simulink subsystem "Pack_SOC_Estimation"  (R2021a)
settings: Solver=VariableStepAuto  StartTime=0.0  StopTime=10.0  RelTol=1e-3
(part 2 of 4)

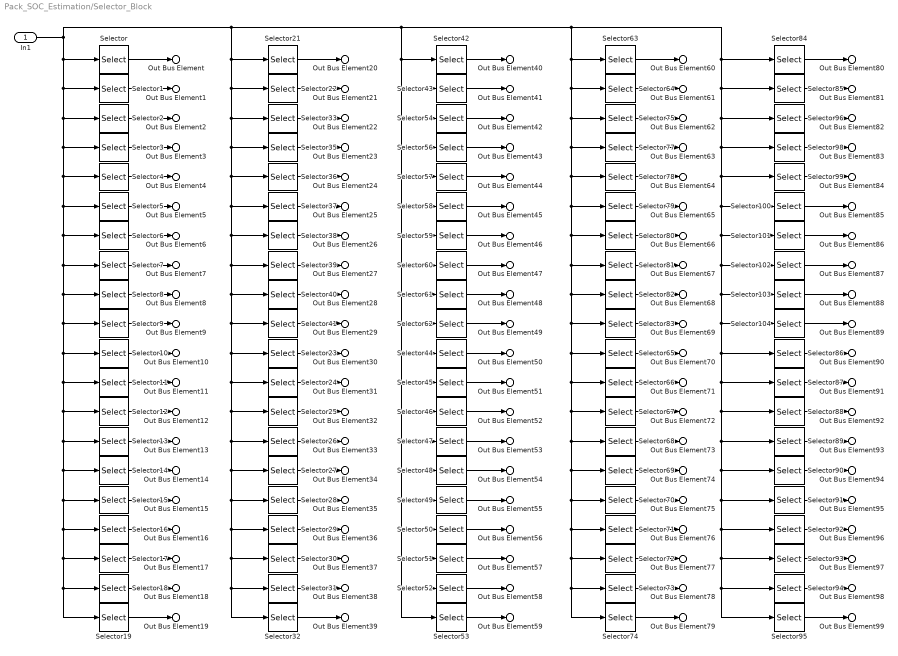
== system Pack_SOC_Estimation/Selector_Block ==
  In1 : Inport
  Selector : Selector  NumberOfDimensions=2  InputPortWidth=3  IndexOptions=Index vector (dialog),Index vector (dialog)  Indices=1,1  OutputSizes=1,1
  Selector1 : Selector  NumberOfDimensions=2  InputPortWidth=3  IndexOptions=Index vector (dialog),Index vector (dialog)  Indices=1,2  OutputSizes=1,1
  Selector10 : Selector  NumberOfDimensions=2  InputPortWidth=3  IndexOptions=Index vector (dialog),Index vector (dialog)  Indices=2,1  OutputSizes=1,1
  Selector100 : Selector  NumberOfDimensions=2  InputPortWidth=3  IndexOptions=Index vector (dialog),Index vector (dialog)  Indices=9,6  OutputSizes=1,1
  Selector101 : Selector  NumberOfDimensions=2  InputPortWidth=3  IndexOptions=Index vector (dialog),Index vector (dialog)  Indices=9,7  OutputSizes=1,1
  Selector102 : Selector  NumberOfDimensions=2  InputPortWidth=3  IndexOptions=Index vector (dialog),Index vector (dialog)  Indices=9,8  OutputSizes=1,1
  Selector103 : Selector  NumberOfDimensions=2  InputPortWidth=3  IndexOptions=Index vector (dialog),Index vector (dialog)  Indices=9,9  OutputSizes=1,1
  Selector104 : Selector  NumberOfDimensions=2  InputPortWidth=3  IndexOptions=Index vector (dialog),Index vector (dialog)  Indices=9,10  OutputSizes=1,1
  Selector11 : Selector  NumberOfDimensions=2  InputPortWidth=3  IndexOptions=Index vector (dialog),Index vector (dialog)  Indices=2,2  OutputSizes=1,1
  Selector12 : Selector  NumberOfDimensions=2  InputPortWidth=3  IndexOptions=Index vector (dialog),Index vector (dialog)  Indices=2,3  OutputSizes=1,1
  Selector13 : Selector  NumberOfDimensions=2  InputPortWidth=3  IndexOptions=Index vector (dialog),Index vector (dialog)  Indices=2,4  OutputSizes=1,1
  Selector14 : Selector  NumberOfDimensions=2  InputPortWidth=3  IndexOptions=Index vector (dialog),Index vector (dialog)  Indices=2,5  OutputSizes=1,1
  Selector15 : Selector  NumberOfDimensions=2  InputPortWidth=3  IndexOptions=Index vector (dialog),Index vector (dialog)  Indices=2,6  OutputSizes=1,1
  Selector16 : Selector  NumberOfDimensions=2  InputPortWidth=3  IndexOptions=Index vector (dialog),Index vector (dialog)  Indices=2,7  OutputSizes=1,1
  Selector17 : Selector  NumberOfDimensions=2  InputPortWidth=3  IndexOptions=Index vector (dialog),Index vector (dialog)  Indices=2,8  OutputSizes=1,1
  Selector18 : Selector  NumberOfDimensions=2  InputPortWidth=3  IndexOptions=Index vector (dialog),Index vector (dialog)  Indices=2,9  OutputSizes=1,1
  Selector19 : Selector  NumberOfDimensions=2  InputPortWidth=3  IndexOptions=Index vector (dialog),Index vector (dialog)  Indices=2,10  OutputSizes=1,1
  Selector2 : Selector  NumberOfDimensions=2  InputPortWidth=3  IndexOptions=Index vector (dialog),Index vector (dialog)  Indices=1,3  OutputSizes=1,1
  Selector21 : Selector  NumberOfDimensions=2  InputPortWidth=3  IndexOptions=Index vector (dialog),Index vector (dialog)  Indices=3,1  OutputSizes=1,1
  Selector22 : Selector  NumberOfDimensions=2  InputPortWidth=3  IndexOptions=Index vector (dialog),Index vector (dialog)  Indices=3,2  OutputSizes=1,1
  Selector23 : Selector  NumberOfDimensions=2  InputPortWidth=3  IndexOptions=Index vector (dialog),Index vector (dialog)  Indices=4,1  OutputSizes=1,1
  Selector24 : Selector  NumberOfDimensions=2  InputPortWidth=3  IndexOptions=Index vector (dialog),Index vector (dialog)  Indices=4,2  OutputSizes=1,1
  Selector25 : Selector  NumberOfDimensions=2  InputPortWidth=3  IndexOptions=Index vector (dialog),Index vector (dialog)  Indices=4,3  OutputSizes=1,1
  Selector26 : Selector  NumberOfDimensions=2  InputPortWidth=3  IndexOptions=Index vector (dialog),Index vector (dialog)  Indices=4,4  OutputSizes=1,1
  Selector27 : Selector  NumberOfDimensions=2  InputPortWidth=3  IndexOptions=Index vector (dialog),Index vector (dialog)  Indices=4,5  OutputSizes=1,1
  Selector28 : Selector  NumberOfDimensions=2  InputPortWidth=3  IndexOptions=Index vector (dialog),Index vector (dialog)  Indices=4,6  OutputSizes=1,1
  Selector29 : Selector  NumberOfDimensions=2  InputPortWidth=3  IndexOptions=Index vector (dialog),Index vector (dialog)  Indices=4,7  OutputSizes=1,1
  Selector3 : Selector  NumberOfDimensions=2  InputPortWidth=3  IndexOptions=Index vector (dialog),Index vector (dialog)  Indices=1,4  OutputSizes=1,1
  Selector30 : Selector  NumberOfDimensions=2  InputPortWidth=3  IndexOptions=Index vector (dialog),Index vector (dialog)  Indices=4,8  OutputSizes=1,1
  Selector31 : Selector  NumberOfDimensions=2  InputPortWidth=3  IndexOptions=Index vector (dialog),Index vector (dialog)  Indices=4,9  OutputSizes=1,1
  Selector32 : Selector  NumberOfDimensions=2  InputPortWidth=3  IndexOptions=Index vector (dialog),Index vector (dialog)  Indices=4,10  OutputSizes=1,1
  Selector33 : Selector  NumberOfDimensions=2  InputPortWidth=3  IndexOptions=Index vector (dialog),Index vector (dialog)  Indices=3,3  OutputSizes=1,1
  Selector35 : Selector  NumberOfDimensions=2  InputPortWidth=3  IndexOptions=Index vector (dialog),Index vector (dialog)  Indices=3,4  OutputSizes=1,1
  Selector36 : Selector  NumberOfDimensions=2  InputPortWidth=3  IndexOptions=Index vector (dialog),Index vector (dialog)  Indices=3,5  OutputSizes=1,1
  Selector37 : Selector  NumberOfDimensions=2  InputPortWidth=3  IndexOptions=Index vector (dialog),Index vector (dialog)  Indices=3,6  OutputSizes=1,1
  Selector38 : Selector  NumberOfDimensions=2  InputPortWidth=3  IndexOptions=Index vector (dialog),Index vector (dialog)  Indices=3,7  OutputSizes=1,1
  Selector39 : Selector  NumberOfDimensions=2  InputPortWidth=3  IndexOptions=Index vector (dialog),Index vector (dialog)  Indices=3,8  OutputSizes=1,1
  Selector4 : Selector  NumberOfDimensions=2  InputPortWidth=3  IndexOptions=Index vector (dialog),Index vector (dialog)  Indices=1,5  OutputSizes=1,1
  Selector40 : Selector  NumberOfDimensions=2  InputPortWidth=3  IndexOptions=Index vector (dialog),Index vector (dialog)  Indices=3,9  OutputSizes=1,1
  Selector41 : Selector  NumberOfDimensions=2  InputPortWidth=3  IndexOptions=Index vector (dialog),Index vector (dialog)  Indices=3,10  OutputSizes=1,1
  Selector42 : Selector  NumberOfDimensions=2  InputPortWidth=3  IndexOptions=Index vector (dialog),Index vector (dialog)  Indices=5,1  OutputSizes=1,1
  Selector43 : Selector  NumberOfDimensions=2  InputPortWidth=3  IndexOptions=Index vector (dialog),Index vector (dialog)  Indices=5,2  OutputSizes=1,1
  Selector44 : Selector  NumberOfDimensions=2  InputPortWidth=3  IndexOptions=Index vector (dialog),Index vector (dialog)  Indices=6,1  OutputSizes=1,1
  Selector45 : Selector  NumberOfDimensions=2  InputPortWidth=3  IndexOptions=Index vector (dialog),Index vector (dialog)  Indices=6,2  OutputSizes=1,1
  Selector46 : Selector  NumberOfDimensions=2  InputPortWidth=3  IndexOptions=Index vector (dialog),Index vector (dialog)  Indices=6,3  OutputSizes=1,1
  Selector47 : Selector  NumberOfDimensions=2  InputPortWidth=3  IndexOptions=Index vector (dialog),Index vector (dialog)  Indices=6,4  OutputSizes=1,1
  Selector48 : Selector  NumberOfDimensions=2  InputPortWidth=3  IndexOptions=Index vector (dialog),Index vector (dialog)  Indices=6,5  OutputSizes=1,1
  Selector49 : Selector  NumberOfDimensions=2  InputPortWidth=3  IndexOptions=Index vector (dialog),Index vector (dialog)  Indices=6,6  OutputSizes=1,1
  Selector5 : Selector  NumberOfDimensions=2  InputPortWidth=3  IndexOptions=Index vector (dialog),Index vector (dialog)  Indices=1,6  OutputSizes=1,1
  Selector50 : Selector  NumberOfDimensions=2  InputPortWidth=3  IndexOptions=Index vector (dialog),Index vector (dialog)  Indices=6,7  OutputSizes=1,1
  Selector51 : Selector  NumberOfDimensions=2  InputPortWidth=3  IndexOptions=Index vector (dialog),Index vector (dialog)  Indices=6,8  OutputSizes=1,1
  Selector52 : Selector  NumberOfDimensions=2  InputPortWidth=3  IndexOptions=Index vector (dialog),Index vector (dialog)  Indices=6,9  OutputSizes=1,1
  Selector53 : Selector  NumberOfDimensions=2  InputPortWidth=3  IndexOptions=Index vector (dialog),Index vector (dialog)  Indices=6,10  OutputSizes=1,1
  Selector54 : Selector  NumberOfDimensions=2  InputPortWidth=3  IndexOptions=Index vector (dialog),Index vector (dialog)  Indices=5,3  OutputSizes=1,1
  Selector56 : Selector  NumberOfDimensions=2  InputPortWidth=3  IndexOptions=Index vector (dialog),Index vector (dialog)  Indices=5,4  OutputSizes=1,1
  Selector57 : Selector  NumberOfDimensions=2  InputPortWidth=3  IndexOptions=Index vector (dialog),Index vector (dialog)  Indices=5,5  OutputSizes=1,1
  Selector58 : Selector  NumberOfDimensions=2  InputPortWidth=3  IndexOptions=Index vector (dialog),Index vector (dialog)  Indices=5,6  OutputSizes=1,1
  Selector59 : Selector  NumberOfDimensions=2  InputPortWidth=3  IndexOptions=Index vector (dialog),Index vector (dialog)  Indices=5,7  OutputSizes=1,1
  Selector6 : Selector  NumberOfDimensions=2  InputPortWidth=3  IndexOptions=Index vector (dialog),Index vector (dialog)  Indices=1,7  OutputSizes=1,1
  Selector60 : Selector  NumberOfDimensions=2  InputPortWidth=3  IndexOptions=Index vector (dialog),Index vector (dialog)  Indices=5,8  OutputSizes=1,1
  Selector61 : Selector  NumberOfDimensions=2  InputPortWidth=3  IndexOptions=Index vector (dialog),Index vector (dialog)  Indices=5,9  OutputSizes=1,1
  Selector62 : Selector  NumberOfDimensions=2  InputPortWidth=3  IndexOptions=Index vector (dialog),Index vector (dialog)  Indices=5,10  OutputSizes=1,1
  Selector63 : Selector  NumberOfDimensions=2  InputPortWidth=3  IndexOptions=Index vector (dialog),Index vector (dialog)  Indices=7,1  OutputSizes=1,1
  Selector64 : Selector  NumberOfDimensions=2  InputPortWidth=3  IndexOptions=Index vector (dialog),Index vector (dialog)  Indices=7,2  OutputSizes=1,1
  Selector65 : Selector  NumberOfDimensions=2  InputPortWidth=3  IndexOptions=Index vector (dialog),Index vector (dialog)  Indices=8,1  OutputSizes=1,1
  Selector66 : Selector  NumberOfDimensions=2  InputPortWidth=3  IndexOptions=Index vector (dialog),Index vector (dialog)  Indices=8,2  OutputSizes=1,1
  Selector67 : Selector  NumberOfDimensions=2  InputPortWidth=3  IndexOptions=Index vector (dialog),Index vector (dialog)  Indices=8,3  OutputSizes=1,1
  Selector68 : Selector  NumberOfDimensions=2  InputPortWidth=3  IndexOptions=Index vector (dialog),Index vector (dialog)  Indices=8,4  OutputSizes=1,1
  Selector69 : Selector  NumberOfDimensions=2  InputPortWidth=3  IndexOptions=Index vector (dialog),Index vector (dialog)  Indices=8,5  OutputSizes=1,1
  Selector7 : Selector  NumberOfDimensions=2  InputPortWidth=3  IndexOptions=Index vector (dialog),Index vector (dialog)  Indices=1,8  OutputSizes=1,1
  Selector70 : Selector  NumberOfDimensions=2  InputPortWidth=3  IndexOptions=Index vector (dialog),Index vector (dialog)  Indices=8,6  OutputSizes=1,1
  Selector71 : Selector  NumberOfDimensions=2  InputPortWidth=3  IndexOptions=Index vector (dialog),Index vector (dialog)  Indices=8,7  OutputSizes=1,1
  Selector72 : Selector  NumberOfDimensions=2  InputPortWidth=3  IndexOptions=Index vector (dialog),Index vector (dialog)  Indices=8,8  OutputSizes=1,1
  Selector73 : Selector  NumberOfDimensions=2  InputPortWidth=3  IndexOptions=Index vector (dialog),Index vector (dialog)  Indices=8,9  OutputSizes=1,1
  Selector74 : Selector  NumberOfDimensions=2  InputPortWidth=3  IndexOptions=Index vector (dialog),Index vector (dialog)  Indices=8,10  OutputSizes=1,1
  Selector75 : Selector  NumberOfDimensions=2  InputPortWidth=3  IndexOptions=Index vector (dialog),Index vector (dialog)  Indices=7,3  OutputSizes=1,1
  Selector77 : Selector  NumberOfDimensions=2  InputPortWidth=3  IndexOptions=Index vector (dialog),Index vector (dialog)  Indices=7,4  OutputSizes=1,1
  Selector78 : Selector  NumberOfDimensions=2  InputPortWidth=3  IndexOptions=Index vector (dialog),Index vector (dialog)  Indices=7,5  OutputSizes=1,1
  Selector79 : Selector  NumberOfDimensions=2  InputPortWidth=3  IndexOptions=Index vector (dialog),Index vector (dialog)  Indices=7,6  OutputSizes=1,1
  Selector8 : Selector  NumberOfDimensions=2  InputPortWidth=3  IndexOptions=Index vector (dialog),Index vector (dialog)  Indices=1,9  OutputSizes=1,1
  Selector80 : Selector  NumberOfDimensions=2  InputPortWidth=3  IndexOptions=Index vector (dialog),Index vector (dialog)  Indices=7,7  OutputSizes=1,1
  Selector81 : Selector  NumberOfDimensions=2  InputPortWidth=3  IndexOptions=Index vector (dialog),Index vector (dialog)  Indices=7,8  OutputSizes=1,1
  Selector82 : Selector  NumberOfDimensions=2  InputPortWidth=3  IndexOptions=Index vector (dialog),Index vector (dialog)  Indices=7,9  OutputSizes=1,1
  Selector83 : Selector  NumberOfDimensions=2  InputPortWidth=3  IndexOptions=Index vector (dialog),Index vector (dialog)  Indices=7,10  OutputSizes=1,1
  Selector84 : Selector  NumberOfDimensions=2  InputPortWidth=3  IndexOptions=Index vector (dialog),Index vector (dialog)  Indices=9,1  OutputSizes=1,1
  Selector85 : Selector  NumberOfDimensions=2  InputPortWidth=3  IndexOptions=Index vector (dialog),Index vector (dialog)  Indices=9,2  OutputSizes=1,1
  Selector86 : Selector  NumberOfDimensions=2  InputPortWidth=3  IndexOptions=Index vector (dialog),Index vector (dialog)  Indices=10,1  OutputSizes=1,1
  Selector87 : Selector  NumberOfDimensions=2  InputPortWidth=3  IndexOptions=Index vector (dialog),Index vector (dialog)  Indices=10,2  OutputSizes=1,1
  Selector88 : Selector  NumberOfDimensions=2  InputPortWidth=3  IndexOptions=Index vector (dialog),Index vector (dialog)  Indices=10,3  OutputSizes=1,1
  Selector89 : Selector  NumberOfDimensions=2  InputPortWidth=3  IndexOptions=Index vector (dialog),Index vector (dialog)  Indices=10,4  OutputSizes=1,1
  Selector9 : Selector  NumberOfDimensions=2  InputPortWidth=3  IndexOptions=Index vector (dialog),Index vector (dialog)  Indices=1,10  OutputSizes=1,1
  Selector90 : Selector  NumberOfDimensions=2  InputPortWidth=3  IndexOptions=Index vector (dialog),Index vector (dialog)  Indices=10,5  OutputSizes=1,1
  Selector91 : Selector  NumberOfDimensions=2  InputPortWidth=3  IndexOptions=Index vector (dialog),Index vector (dialog)  Indices=10,6  OutputSizes=1,1
  Selector92 : Selector  NumberOfDimensions=2  InputPortWidth=3  IndexOptions=Index vector (dialog),Index vector (dialog)  Indices=10,7  OutputSizes=1,1
  Selector93 : Selector  NumberOfDimensions=2  InputPortWidth=3  IndexOptions=Index vector (dialog),Index vector (dialog)  Indices=10,8  OutputSizes=1,1
  Selector94 : Selector  NumberOfDimensions=2  InputPortWidth=3  IndexOptions=Index vector (dialog),Index vector (dialog)  Indices=10,9  OutputSizes=1,1
  Selector95 : Selector  NumberOfDimensions=2  InputPortWidth=3  IndexOptions=Index vector (dialog),Index vector (dialog)  Indices=10,10  OutputSizes=1,1
  Selector96 : Selector  NumberOfDimensions=2  InputPortWidth=3  IndexOptions=Index vector (dialog),Index vector (dialog)  Indices=9,3  OutputSizes=1,1
  Selector98 : Selector  NumberOfDimensions=2  InputPortWidth=3  IndexOptions=Index vector (dialog),Index vector (dialog)  Indices=9,4  OutputSizes=1,1
  Selector99 : Selector  NumberOfDimensions=2  InputPortWidth=3  IndexOptions=Index vector (dialog),Index vector (dialog)  Indices=9,5  OutputSizes=1,1
  Out Bus Element : Outport  PortName=OutBus  Element=Current
  Out Bus Element1 : Outport  PortName=OutBus  Element=signal2
  Out Bus Element2 : Outport  PortName=OutBus  Element=signal3
  Out Bus Element3 : Outport  PortName=OutBus  Element=signal4
  Out Bus Element4 : Outport  PortName=OutBus  Element=signal5
  Out Bus Element5 : Outport  PortName=OutBus  Element=signal6
  Out Bus Element6 : Outport  PortName=OutBus  Element=signal7
  Out Bus Element7 : Outport  PortName=OutBus  Element=signal8
  Out Bus Element8 : Outport  PortName=OutBus  Element=signal9
  Out Bus Element9 : Outport  PortName=OutBus  Element=signal10
  Out Bus Element10 : Outport  PortName=OutBus  Element=signal11
  Out Bus Element11 : Outport  PortName=OutBus  Element=signal12
  Out Bus Element12 : Outport  PortName=OutBus  Element=signal13
  Out Bus Element13 : Outport  PortName=OutBus  Element=signal14
  Out Bus Element14 : Outport  PortName=OutBus  Element=signal15
  Out Bus Element15 : Outport  PortName=OutBus  Element=signal16
  Out Bus Element16 : Outport  PortName=OutBus  Element=signal17
  Out Bus Element17 : Outport  PortName=OutBus  Element=signal18
  Out Bus Element18 : Outport  PortName=OutBus  Element=signal19
  Out Bus Element19 : Outport  PortName=OutBus  Element=signal20
  Out Bus Element20 : Outport  PortName=OutBus  Element=signal21
  Out Bus Element21 : Outport  PortName=OutBus  Element=signal22
  Out Bus Element22 : Outport  PortName=OutBus  Element=signal23
  Out Bus Element23 : Outport  PortName=OutBus  Element=signal24
  Out Bus Element24 : Outport  PortName=OutBus  Element=signal25
  Out Bus Element25 : Outport  PortName=OutBus  Element=signal26
  Out Bus Element26 : Outport  PortName=OutBus  Element=signal27
  Out Bus Element27 : Outport  PortName=OutBus  Element=signal28
  Out Bus Element28 : Outport  PortName=OutBus  Element=signal29
  Out Bus Element29 : Outport  PortName=OutBus  Element=signal30
  Out Bus Element30 : Outport  PortName=OutBus  Element=signal31
  Out Bus Element31 : Outport  PortName=OutBus  Element=signal32
  Out Bus Element32 : Outport  PortName=OutBus  Element=signal33
  Out Bus Element33 : Outport  PortName=OutBus  Element=signal34
  Out Bus Element34 : Outport  PortName=OutBus  Element=signal35
  Out Bus Element35 : Outport  PortName=OutBus  Element=signal36
  Out Bus Element36 : Outport  PortName=OutBus  Element=signal37
  Out Bus Element37 : Outport  PortName=OutBus  Element=signal38
  Out Bus Element38 : Outport  PortName=OutBus  Element=signal39
  Out Bus Element39 : Outport  PortName=OutBus  Element=signal40
  Out Bus Element40 : Outport  PortName=OutBus  Element=signal41
  Out Bus Element41 : Outport  PortName=OutBus  Element=signal42
  Out Bus Element42 : Outport  PortName=OutBus  Element=signal43
  Out Bus Element43 : Outport  PortName=OutBus  Element=signal44
  Out Bus Element44 : Outport  PortName=OutBus  Element=signal45
  Out Bus Element45 : Outport  PortName=OutBus  Element=signal46
  Out Bus Element46 : Outport  PortName=OutBus  Element=signal47
  Out Bus Element47 : Outport  PortName=OutBus  Element=signal48
  Out Bus Element48 : Outport  PortName=OutBus  Element=signal49
  Out Bus Element49 : Outport  PortName=OutBus  Element=signal50
  Out Bus Element50 : Outport  PortName=OutBus  Element=signal51
  Out Bus Element51 : Outport  PortName=OutBus  Element=signal52
  Out Bus Element52 : Outport  PortName=OutBus  Element=signal53
  Out Bus Element53 : Outport  PortName=OutBus  Element=signal54
  Out Bus Element54 : Outport  PortName=OutBus  Element=signal55
  Out Bus Element55 : Outport  PortName=OutBus  Element=signal56
  Out Bus Element56 : Outport  PortName=OutBus  Element=signal57
  Out Bus Element57 : Outport  PortName=OutBus  Element=signal58
  Out Bus Element58 : Outport  PortName=OutBus  Element=signal59
  Out Bus Element59 : Outport  PortName=OutBus  Element=signal60
  Out Bus Element60 : Outport  PortName=OutBus  Element=signal61
  Out Bus Element61 : Outport  PortName=OutBus  Element=signal62
  Out Bus Element62 : Outport  PortName=OutBus  Element=signal63
  Out Bus Element63 : Outport  PortName=OutBus  Element=signal64
  Out Bus Element64 : Outport  PortName=OutBus  Element=signal65
  Out Bus Element65 : Outport  PortName=OutBus  Element=signal66
  Out Bus Element66 : Outport  PortName=OutBus  Element=signal67
  Out Bus Element67 : Outport  PortName=OutBus  Element=signal68
  Out Bus Element68 : Outport  PortName=OutBus  Element=signal69
  Out Bus Element69 : Outport  PortName=OutBus  Element=signal70
  Out Bus Element70 : Outport  PortName=OutBus  Element=signal71
  Out Bus Element71 : Outport  PortName=OutBus  Element=signal72
  Out Bus Element72 : Outport  PortName=OutBus  Element=signal73
  Out Bus Element73 : Outport  PortName=OutBus  Element=signal74
  Out Bus Element74 : Outport  PortName=OutBus  Element=signal75
  Out Bus Element75 : Outport  PortName=OutBus  Element=signal76
  Out Bus Element76 : Outport  PortName=OutBus  Element=signal77
  Out Bus Element77 : Outport  PortName=OutBus  Element=signal78
  Out Bus Element78 : Outport  PortName=OutBus  Element=signal79
  Out Bus Element79 : Outport  PortName=OutBus  Element=signal80
  Out Bus Element80 : Outport  PortName=OutBus  Element=signal81
  Out Bus Element81 : Outport  PortName=OutBus  Element=signal82
  Out Bus Element82 : Outport  PortName=OutBus  Element=signal83
  Out Bus Element83 : Outport  PortName=OutBus  Element=signal84
  Out Bus Element84 : Outport  PortName=OutBus  Element=signal85
  Out Bus Element85 : Outport  PortName=OutBus  Element=signal86
  Out Bus Element86 : Outport  PortName=OutBus  Element=signal87
  Out Bus Element87 : Outport  PortName=OutBus  Element=signal88
  Out Bus Element88 : Outport  PortName=OutBus  Element=signal89
  Out Bus Element89 : Outport  PortName=OutBus  Element=signal90
  Out Bus Element90 : Outport  PortName=OutBus  Element=signal91
  Out Bus Element91 : Outport  PortName=OutBus  Element=signal92
  Out Bus Element92 : Outport  PortName=OutBus  Element=signal93
  Out Bus Element93 : Outport  PortName=OutBus  Element=signal94
  Out Bus Element94 : Outport  PortName=OutBus  Element=signal95
  Out Bus Element95 : Outport  PortName=OutBus  Element=signal96
  Out Bus Element96 : Outport  PortName=OutBus  Element=signal97
  Out Bus Element97 : Outport  PortName=OutBus  Element=signal98
  Out Bus Element98 : Outport  PortName=OutBus  Element=signal99
  Out Bus Element99 : Outport  PortName=OutBus  Element=signal100
  wires:
  Selector102/1 -> Out Bus Element87/1
  Selector101/1 -> Out Bus Element86/1
  Selector87/1 -> Out Bus Element91/1
  Selector91/1 -> Out Bus Element95/1
  Selector99/1 -> Out Bus Element84/1
  Selector86/1 -> Out Bus Element90/1
  Selector104/1 -> Out Bus Element89/1
  Selector100/1 -> Out Bus Element85/1
  Selector84/1 -> Out Bus Element80/1
  Selector96/1 -> Out Bus Element82/1
  Selector98/1 -> Out Bus Element83/1
  Selector85/1 -> Out Bus Element81/1
  Selector103/1 -> Out Bus Element88/1
  Selector95/1 -> Out Bus Element99/1
  Selector94/1 -> Out Bus Element98/1
  Selector88/1 -> Out Bus Element92/1
  Selector90/1 -> Out Bus Element94/1
  Selector89/1 -> Out Bus Element93/1
  Selector93/1 -> Out Bus Element97/1
  Selector92/1 -> Out Bus Element96/1
  Selector81/1 -> Out Bus Element67/1
  Selector80/1 -> Out Bus Element66/1
  Selector66/1 -> Out Bus Element71/1
  Selector70/1 -> Out Bus Element75/1
  Selector78/1 -> Out Bus Element64/1
  Selector65/1 -> Out Bus Element70/1
  Selector83/1 -> Out Bus Element69/1
  Selector79/1 -> Out Bus Element65/1
  Selector63/1 -> Out Bus Element60/1
  Selector75/1 -> Out Bus Element62/1
  Selector77/1 -> Out Bus Element63/1
  Selector64/1 -> Out Bus Element61/1
  Selector82/1 -> Out Bus Element68/1
  Selector74/1 -> Out Bus Element79/1
  Selector73/1 -> Out Bus Element78/1
  Selector67/1 -> Out Bus Element72/1
  Selector69/1 -> Out Bus Element74/1
  Selector68/1 -> Out Bus Element73/1
  Selector72/1 -> Out Bus Element77/1
  Selector71/1 -> Out Bus Element76/1
  Selector60/1 -> Out Bus Element47/1
  Selector59/1 -> Out Bus Element46/1
  Selector45/1 -> Out Bus Element51/1
  Selector49/1 -> Out Bus Element55/1
  Selector57/1 -> Out Bus Element44/1
  Selector44/1 -> Out Bus Element50/1
  Selector62/1 -> Out Bus Element49/1
  Selector58/1 -> Out Bus Element45/1
  Selector42/1 -> Out Bus Element40/1
  Selector54/1 -> Out Bus Element42/1
  Selector56/1 -> Out Bus Element43/1
  Selector43/1 -> Out Bus Element41/1
  Selector61/1 -> Out Bus Element48/1
  Selector53/1 -> Out Bus Element59/1
  Selector52/1 -> Out Bus Element58/1
  Selector46/1 -> Out Bus Element52/1
  Selector48/1 -> Out Bus Element54/1
  Selector47/1 -> Out Bus Element53/1
  Selector51/1 -> Out Bus Element57/1
  Selector50/1 -> Out Bus Element56/1
  Selector39/1 -> Out Bus Element27/1
  Selector38/1 -> Out Bus Element26/1
  Selector24/1 -> Out Bus Element31/1
  Selector28/1 -> Out Bus Element35/1
  Selector36/1 -> Out Bus Element24/1
  Selector23/1 -> Out Bus Element30/1
  Selector41/1 -> Out Bus Element29/1
  Selector37/1 -> Out Bus Element25/1
  Selector21/1 -> Out Bus Element20/1
  Selector33/1 -> Out Bus Element22/1
  Selector35/1 -> Out Bus Element23/1
  Selector22/1 -> Out Bus Element21/1
  Selector40/1 -> Out Bus Element28/1
  Selector32/1 -> Out Bus Element39/1
  Selector31/1 -> Out Bus Element38/1
  Selector25/1 -> Out Bus Element32/1
  Selector27/1 -> Out Bus Element34/1
  Selector26/1 -> Out Bus Element33/1
  Selector30/1 -> Out Bus Element37/1
  Selector29/1 -> Out Bus Element36/1
  Selector17/1 -> Out Bus Element17/1
  Selector16/1 -> Out Bus Element16/1
  Selector14/1 -> Out Bus Element14/1
  Selector19/1 -> Out Bus Element19/1
  Selector15/1 -> Out Bus Element15/1
  Selector10/1 -> Out Bus Element10/1
  Selector12/1 -> Out Bus Element12/1
  Selector13/1 -> Out Bus Element13/1
  Selector11/1 -> Out Bus Element11/1
  Selector18/1 -> Out Bus Element18/1
  Selector7/1 -> Out Bus Element7/1
  Selector5/1 -> Out Bus Element5/1
  Selector8/1 -> Out Bus Element8/1
  Selector9/1 -> Out Bus Element9/1
  Selector6/1 -> Out Bus Element6/1
  Selector4/1 -> Out Bus Element4/1
  Selector3/1 -> Out Bus Element3/1
  Selector2/1 -> Out Bus Element2/1
  Selector1/1 -> Out Bus Element1/1
  In1/1 -> Selector/1, Selector18/1, Selector19/1, Selector17/1, Selector16/1, Selector15/1, Selector14/1, Selector13/1, Selector12/1, Selector11/1, Selector10/1, Selector9/1, Selector8/1, Selector7/1, Selector6/1, Selector5/1, Selector4/1, Selector3/1, Selector2/1, Selector1/1, Selector21/1, Selector32/1, Selector31/1, Selector30/1, Selector29/1, Selector28/1, Selector27/1, Selector26/1, Selector25/1, Selector24/1, Selector23/1, Selector41/1, Selector40/1, Selector39/1, Selector38/1, Selector37/1, Selector36/1, Selector35/1, Selector33/1, Selector22/1, Selector42/1, Selector43/1, Selector53/1, Selector52/1, Selector51/1, Selector50/1, Selector49/1, Selector48/1, Selector47/1, Selector46/1, Selector45/1, Selector44/1, Selector62/1, Selector61/1, Selector60/1, Selector59/1, Selector58/1, Selector57/1, Selector56/1, Selector54/1, Selector74/1, Selector73/1, Selector72/1, Selector71/1, Selector70/1, Selector69/1, Selector68/1, Selector67/1, Selector66/1, Selector65/1, Selector83/1, Selector82/1, Selector81/1, Selector80/1, Selector79/1, Selector78/1, Selector77/1, Selector75/1, Selector64/1, Selector63/1, Selector84/1, Selector95/1, Selector94/1, Selector93/1, Selector92/1, Selector91/1, Selector90/1, Selector89/1, Selector88/1, Selector87/1, Selector86/1, Selector104/1, Selector103/1, Selector102/1, Selector101/1, Selector100/1, Selector99/1, Selector98/1, Selector96/1, Selector85/1
  Selector/1 -> Out Bus Element/1
